simulink model "untitled3"  (R2018b)
settings: Solver=VariableStepAuto  StartTime=0.0  StopTime=5  RelTol=1e-3
libraries: commutil2 x4, dspquant2 x4, dsparch4 x2, dspsigops x2, dspindex x1
settings Model: Creator=nhat  LastModifiedBy=nhat

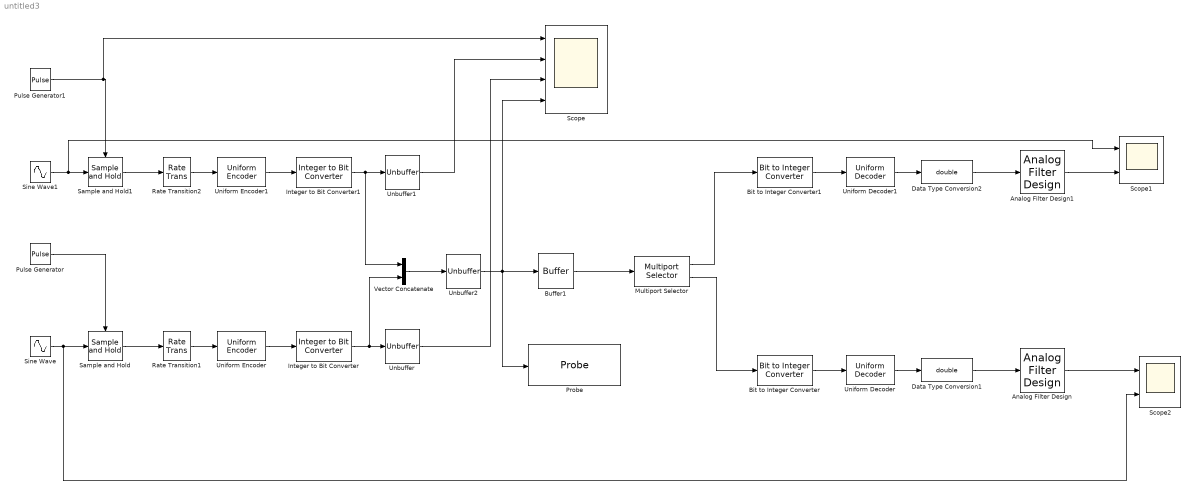
== system untitled3 ==
  Analog Filter Design : dsparch4/Analog Filter Design  method=Butterworth  filttype=Lowpass  N=8  Wlo=3100*2*pi  Whi=80  Rp=2  Rs=40
  Analog Filter Design1 : dsparch4/Analog Filter Design  method=Butterworth  filttype=Lowpass  N=8  Wlo=3100*2*pi  Whi=80  Rp=2  Rs=40
  Bit to Integer Converter : commutil2/Bit to Integer Converter  nbits=8  bitOrder=MSB first  signedOutputValues=Unsigned  outDtype=Inherit via internal rule  outDtypeSigned=Inherit via internal rule
  Bit to Integer Converter1 : commutil2/Bit to Integer Converter  nbits=8  bitOrder=MSB first  signedOutputValues=Unsigned  outDtype=Inherit via internal rule  outDtypeSigned=Inherit via internal rule
  Buffer1 : Buffer  N=16  OutputFrames=off
  Data Type Conversion1 : DataTypeConversion  OutDataTypeStr=double
  Data Type Conversion2 : DataTypeConversion  OutDataTypeStr=double
  Integer to Bit Converter : commutil2/Integer to Bit Converter  nbits=8  signedInputValues=Unsigned  bitOrder=MSB first  outDtype=Inherit via internal rule
  Integer to Bit Converter1 : commutil2/Integer to Bit Converter  nbits=8  signedInputValues=Unsigned  bitOrder=MSB first  outDtype=Inherit via internal rule
  Multiport Selector : dspindex/Multiport Selector  rowsOrCols=Rows  idxCellArray={ [1:8], [9: 16] }  idxErrMode=Clip Index
  Probe : Probe  ProbeSignalDimensions=on  ProbeWidthDataType=Same as input  ProbeSampleTimeDataType=Same as input  ProbeComplexityDataType=Same as input  ProbeDimensionsDataType=Same as input
  Pulse Generator : DiscretePulseGenerator  PulseType=Time based  Period=1/8000  PulseWidth=50
  Pulse Generator1 : DiscretePulseGenerator  PulseType=Time based  Period=1/8000  PulseWidth=50
  Rate Transition1 : RateTransition  OutPortSampleTime=1/8000
  Rate Transition2 : RateTransition  OutPortSampleTime=1/8000
  Sample and Hold : dspsigops/Sample and Hold  trig=Rising edge  initCond=0  latchinput=off
  Sample and Hold1 : dspsigops/Sample and Hold  trig=Rising edge  initCond=0  latchinput=off
  Scope : Scope  NumInputPorts=4
  Scope1 : Scope  NumInputPorts=2
  Scope2 : Scope  NumInputPorts=2
  Sine Wave : Sin  Frequency=3000*2*pi  SampleTime=1/64000
  Sine Wave1 : Sin  Frequency=3000*2*pi  SampleTime=1/64000
  Unbuffer : Unbuffer
  Unbuffer1 : Unbuffer
  Unbuffer2 : Unbuffer
  Uniform Decoder : dspquant2/Uniform Decoder  peak=1  bits=8  overflowMode=Saturate  otype=Double
      settings: SourceProductName=DSP System Toolbox  SourceProductBaseCode=DS
  Uniform Decoder1 : dspquant2/Uniform Decoder  peak=1  bits=8  overflowMode=Saturate  otype=Double
      settings: SourceProductName=DSP System Toolbox  SourceProductBaseCode=DS
  Uniform Encoder : dspquant2/Uniform Encoder  peak=1  bits=8  otype=Unsigned integer
      settings: SourceProductName=DSP System Toolbox
  Uniform Encoder1 : dspquant2/Uniform Encoder  peak=1  bits=8  otype=Unsigned integer
      settings: SourceProductName=DSP System Toolbox
  Vector Concatenate : Concatenate
  wires:
  Bit to Integer Converter/1 -> Uniform Decoder/1
  Uniform Encoder/1 -> Integer to Bit Converter/1
  Integer to Bit Converter/1 -> Vector Concatenate/2, Unbuffer/1
  Rate Transition1/1 -> Uniform Encoder/1
  Sample and Hold/1 -> Rate Transition1/1
  Pulse Generator/1 -> Sample and Hold/Trigger
  Sine Wave/1 -> Scope2/2, Sample and Hold/1
  Multiport Selector/2 -> Bit to Integer Converter/1
  Uniform Decoder/1 -> Data Type Conversion1/1
  Data Type Conversion1/1 -> Analog Filter Design/1
  Sample and Hold1/1 -> Rate Transition2/1
  Integer to Bit Converter1/1 -> Vector Concatenate/1, Unbuffer1/1
  Pulse Generator1/1 -> Scope/1, Sample and Hold1/Trigger
  Rate Transition2/1 -> Uniform Encoder1/1
  Uniform Encoder1/1 -> Integer to Bit Converter1/1
  Sine Wave1/1 -> Scope1/1, Sample and Hold1/1
  Vector Concatenate/1 -> Unbuffer2/1
  Unbuffer2/1 -> Scope/4, Probe/1, Buffer1/1
  Buffer1/1 -> Multiport Selector/1
  Unbuffer/1 -> Scope/3
  Unbuffer1/1 -> Scope/2
  Uniform Decoder1/1 -> Data Type Conversion2/1
  Data Type Conversion2/1 -> Analog Filter Design1/1
  Multiport Selector/1 -> Bit to Integer Converter1/1
  Bit to Integer Converter1/1 -> Uniform Decoder1/1
  Analog Filter Design1/1 -> Scope1/2
  Analog Filter Design/1 -> Scope2/1
